simulink model "SVPWM"  (R2015a)
settings: Solver=ode4  StartTime=0.0  StopTime=40e-3  FixedStep=Ts  RelTol=1e-3
PreLoadFcn:
  | setup;
values from neighbouring files (symbols this model uses):
  Ts = 1e-8    (= 1e-08)    [setup.m]
libraries: powerlib x5, simulink x3
settings Model: CovSFcnEnable=off  Creator=mikaczma  LastModifiedBy=Michał
settings DataIOCC: SaveOutput=off  SaveTime=off
settings DebuggingCC: SolverPrmCheckMsg=warning
settings HardwareCC: ProdHWDeviceType=ASIC/FPGA->ASIC/FPGA  TargetLongLongMode=on  TargetIntDivRoundTo=Zero  TargetEndianess=LittleEndian  TargetHWDeviceType=Generic->MATLAB Host Computer  ProdEqTarget=off

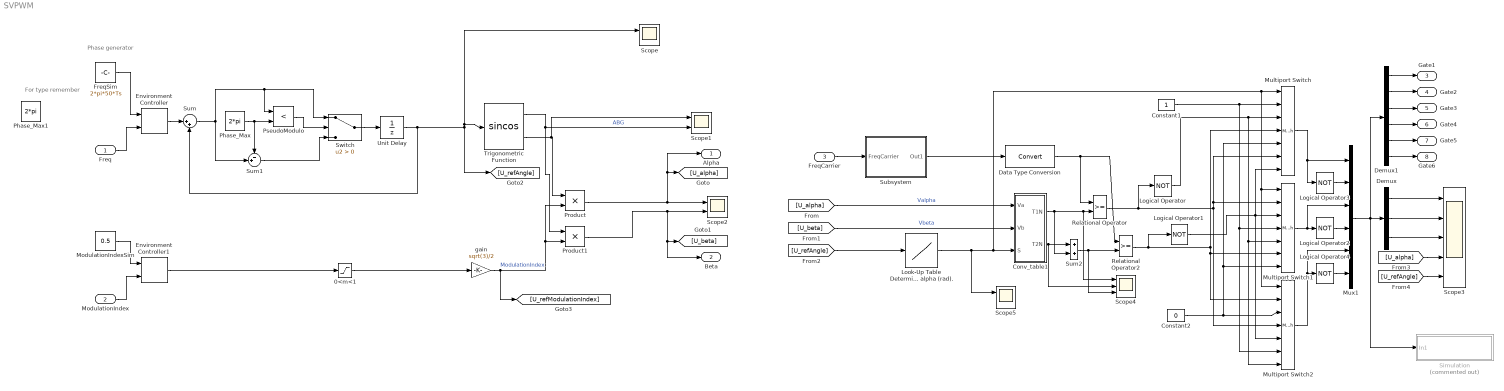
== system SVPWM ==
  note: For type remember
  note: Phase generator
  Freq : Inport
  ModulationIndex : Inport  Port=2
  FreqCarrier : Inport  Port=3
  "0<m<1 " : Saturate  UpperLimit=1  LowerLimit=0
  Constant1 : Constant  OutDataTypeStr=boolean  SampleTime=Ts
  Constant2 : Constant  Value=0  OutDataTypeStr=boolean  SampleTime=Ts
  Conv_table1 : Subsystem  VariantControl=Variant1
  Data Type Conversion : DataTypeConversion
  Demux : Demux  Outputs=[2 2 2]
  Demux1 : Demux  Outputs=6
  Environment Controller : simulink/Signal Routing/Environment Controller
  Environment Controller1 : simulink/Signal Routing/Environment Controller
  FreqSim : Constant  Value=2*pi*50*Ts  OutDataTypeStr=fixdt(1,32,24)  SampleTime=-1
  Logical Operator{,1..4} (5 alike) : Logic  Operator=NOT  OutDataTypeStr=boolean
  "Look-Up Table Determine the sector of U* based on alpha (rad). " : Lookup  InputValues=[0:pi/3:5*pi/3]  Table=[1:6]  LookUpMeth=Use Input Below  SaturateOnIntegerOverflow=on
  ModulationIndexSim : Constant  Value=0.5  OutDataTypeStr=fixdt(1,32,24)  SampleTime=-1
  Multiport Switch : MultiPortSwitch  Inputs=6  SaturateOnIntegerOverflow=on  InputSameDT=on
  Multiport Switch1 : MultiPortSwitch  Inputs=6  SaturateOnIntegerOverflow=on  InputSameDT=on
  Multiport Switch2 : MultiPortSwitch  Inputs=6  SaturateOnIntegerOverflow=on  InputSameDT=on
  Mux1 : Mux  Inputs=6
  Phase_Max : Constant  Value=2*pi  OutDataTypeStr=fixdt(1,32,24)  SampleTime=-1
  Phase_Max1 : Constant  Value=2*pi  OutDataTypeStr=fixdt(1,32,24)  SampleTime=-1
  Product : Product  OutMin=-2  OutMax=2  OutDataTypeStr=fixdt(1,64,60)
  Product1 : Product  OutMin=-2  OutMax=2  OutDataTypeStr=fixdt(1,64,60)
  PseudoModulo : RelationalOperator  Operator=<  OutDataTypeStr=boolean
  Relational Operator : RelationalOperator  OutDataTypeStr=boolean  InputSameDT=on
  Relational Operator2 : RelationalOperator  OutDataTypeStr=boolean  InputSameDT=on
  Scope{,1..2,5} (4 alike) : Scope  NumInputPorts=2
      Scope settings: YMin=0.075~-1  YMax=0.135~1
      Scope1 settings: YMin=-1~-1  YMax=1~1
      Scope2 settings: YMin=-0.45~-0.45  YMax=0.45~0.45  SaveName=ScopeData2
      Scope5 settings: YMin=0.2~-1  YMax=0.4~1  SaveName=ScopeData5
  Scope3 : Scope  NumInputPorts=5
      settings: YMin=0~0~0~-0.4~0  YMax=1~1~1~0.5~2.5  SaveName=ScopeData3
  Scope4 : Scope  NumInputPorts=3
      settings: YMin=-1~-0.5~-5  YMax=0.4~1~5  SaveName=ScopeData4
  Simulation : Subsystem  Commented=on
  Subsystem : Subsystem
  Sum : Sum  Inputs=|++  OutDataTypeStr=Inherit: Same as first input
  Sum1 : Sum  Inputs=-+|  OutMin=0  OutMax=2*pi  OutDataTypeStr=Inherit: Same as first input
  Sum2 : Sum  SaturateOnIntegerOverflow=on  InputSameDT=on  OutDataTypeStr=Inherit: Same as first input
  Switch : Switch  Criteria=u2 > Threshold
  Trigonometric Function : Trigonometry  Operator=sincos  ApproximationMethod=CORDIC  NumberOfIterations=20
  Unit Delay : UnitDelay  SampleTime=-1
  gain : Gain  Gain=sqrt(3)/2  OutDataTypeStr=fixdt(1,32,30)  SaturateOnIntegerOverflow=on  ParamDataTypeStr=Inherit: Same as input
  Alpha : Outport  OutMin=-2  OutMax=2
  Beta : Outport  Port=2  OutMin=-2  OutMax=2
  Gate1 : Outport  Port=3  OutDataTypeStr=boolean
  Gate2 : Outport  Port=4  OutDataTypeStr=boolean
  Gate3 : Outport  Port=5  OutDataTypeStr=boolean
  Gate4 : Outport  Port=6  OutDataTypeStr=boolean
  Gate5 : Outport  Port=7  OutDataTypeStr=boolean
  Gate6 : Outport  Port=8  OutDataTypeStr=boolean
  wires:
  Sum/1 -> Sum1/2, PseudoModulo/1, Switch/1
  Unit Delay/1 -> Trigonometric Function/1, Scope/1, [U_refAngle], Sum/2
  Phase_Max/1 -> PseudoModulo/2, Sum1/1
  PseudoModulo/1 -> Switch/2
  Switch/1 -> Unit Delay/1
  Sum1/1 -> Switch/3
  Environment Controller/1 -> Sum/1
  Freq/1 -> Environment Controller/2
  FreqSim/1 -> Environment Controller/1
  Trigonometric Function/2 -> Scope1/1, Product/1
  ModulationIndex/1 -> Environment Controller1/2
  ModulationIndexSim/1 -> Environment Controller1/1
  Environment Controller1/1 -> "0<m<1 "/1
  Trigonometric Function/1 -> Product1/1, Scope1/2  "ABG"
  "0<m<1 "/1 -> gain/1
  Subsystem/1(Out1) -> Data Type Conversion/1
  [U_beta] -> Conv_table1/2(Vb)  "Vbeta"
  [U_alpha] -> Conv_table1/1(Va)  "Valpha"
  Constant2/1 -> Multiport Switch1/7, Multiport Switch/5, Multiport Switch2/3
  Logical Operator1/1 -> Multiport Switch/7, Multiport Switch2/5, Multiport Switch1/3
  Logical Operator/1 -> Multiport Switch2/7, Multiport Switch1/5, Multiport Switch/3
  Relational Operator2/1 -> Multiport Switch1/6, Multiport Switch2/2, Multiport Switch/4, Logical Operator1/1
  Relational Operator/1 -> Multiport Switch/6, Multiport Switch1/2, Multiport Switch2/4, Logical Operator/1
  Constant1/1 -> Multiport Switch2/6, Multiport Switch1/4, Multiport Switch/2
  Sum2/1 -> Scope4/3, Relational Operator2/2
  Conv_table1/2(T2N) -> Scope4/2, Sum2/1
  Conv_table1/1(T1N) -> Sum2/2, Scope4/1, Relational Operator/2
  Logical Operator3/1 -> Mux1/2
  Logical Operator2/1 -> Mux1/4
  Logical Operator4/1 -> Mux1/6
  Multiport Switch/1 -> Logical Operator3/1, Mux1/1
  Multiport Switch1/1 -> Logical Operator2/1, Mux1/3
  Multiport Switch2/1 -> Mux1/5, Logical Operator4/1
  "Look-Up Table Determine the sector of U* based on alpha (rad). "/1 -> Scope5/1, Conv_table1/3(S), Multiport Switch2/1, Multiport Switch1/1, Multiport Switch/1
  Product/1 -> Alpha/1, [U_alpha], Scope2/1
  Product1/1 -> Beta/1, [U_beta], Scope2/2
  gain/1 -> [U_refModulationIndex], Product1/2, Product/2  "ModulationIndex"
  [U_refAngle] -> "Look-Up Table Determine the sector of U* based on alpha (rad). "/1
  Demux/2 -> Scope3/2
  Demux/1 -> Scope3/1
  Demux/3 -> Scope3/3
  [U_alpha] -> Scope3/4
  [U_refAngle] -> Scope3/5
  Mux1/1 -> Demux1/1, Simulation/1(In1), Demux/1
  Data Type Conversion/1 -> Relational Operator/1, Relational Operator2/1
  Demux1/1 -> Gate1/1
  Demux1/4 -> Gate4/1
  Demux1/3 -> Gate3/1
  Demux1/2 -> Gate2/1
  Demux1/5 -> Gate5/1
  Demux1/6 -> Gate6/1
  FreqCarrier/1 -> Subsystem/1(FreqCarrier)

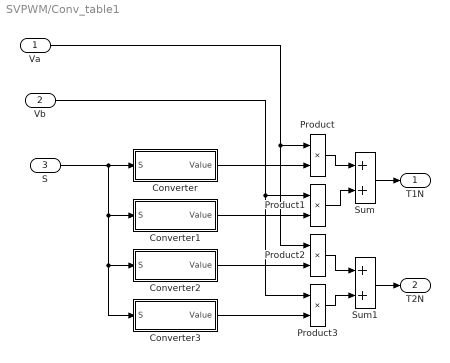
== system SVPWM/Conv_table1 ==
  Va : Inport
  Vb : Inport  Port=2
  S : Inport  Port=3
  Converter : Subsystem  VariantControl=Variant1  mask{Data=[1 1 0 -1 -1 0]}
      mask prompts: Data "Data Coefficients"
      mask Display:
      | port_label('input', 1, 'Sector')
      | port_label('output', 1, 'Value')
  Converter1 : Subsystem  VariantControl=Variant1  mask{Data=[-1/sqrt(3) 1/sqrt(3) 2/sqrt(3) 1/sqrt(3) -1/sqrt(3) -2/sqrt(3)]}
      mask prompts: Data "Data Coefficients"
      mask Display:
      | port_label('input', 1, 'Sector')
      | port_label('output', 1, 'Value')
  Converter2 : Subsystem  VariantControl=Variant1  mask{Data=[0 -1 -1 0 1 1]}
      mask prompts: Data "Data Coefficients"
      mask Display:
      | port_label('input', 1, 'Sector')
      | port_label('output', 1, 'Value')
  Converter3 : Subsystem  VariantControl=Variant1  mask{Data=[2/sqrt(3) 1/sqrt(3) -1/sqrt(3) -2/sqrt(3) -1/sqrt(3) 1/sqrt(3)]}
      mask prompts: Data "Data Coefficients"
      mask Display:
      | port_label('input', 1, 'Sector')
      | port_label('output', 1, 'Value')
  Product{,1..3} (4 alike) : Product  SaturateOnIntegerOverflow=on  InputSameDT=on  OutDataTypeStr=Inherit: Same as first input
  Sum : Sum  SaturateOnIntegerOverflow=on  InputSameDT=on  OutDataTypeStr=Inherit: Same as first input
  Sum1 : Sum  SaturateOnIntegerOverflow=on  InputSameDT=on  OutDataTypeStr=Inherit: Same as first input
  T1N : Outport
  T2N : Outport  Port=2
  wires:
  Va/1 -> Product/1, Product2/1
  Converter/1(Value) -> Product/2
  Vb/1 -> Product1/1, Product3/1
  Converter1/1(Value) -> Product1/2
  Converter2/1(Value) -> Product2/2
  Converter3/1(Value) -> Product3/2
  Product/1 -> Sum/1
  Product1/1 -> Sum/2
  Product2/1 -> Sum1/1
  Product3/1 -> Sum1/2
  Sum/1 -> T1N/1
  Sum1/1 -> T2N/1
  S/1 -> Converter3/1(S), Converter2/1(S), Converter1/1(S), Converter/1(S)

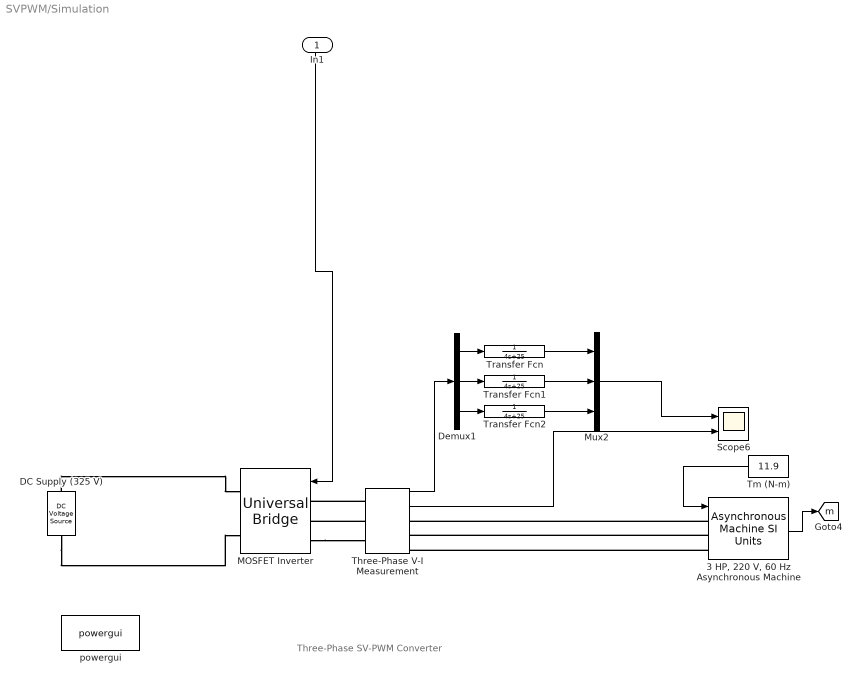
== system SVPWM/Simulation ==
  note: Three-Phase SV-PWM Converter
  In1 : Inport
  "3 HP, 220 V, 60 Hz Asynchronous Machine" : powerlib/Machines/Asynchronous Machine SI Units  RotorType=Squirrel-cage  PresetModel=No  MechanicalLoad=Torque Tm  ShowDetailedParameters=on  ReferenceFrame=Stationary  Units=SI  MeasurementBus=off  NominalParameters=[ 3*746, 220, 60 ]  Stator="[ 0.435  2*2.0e-3 ]"  Rotor="[ 0.816  2.0e-3 ]"  Cage1=[ 0.022 0.226/377]  Cage2=[ 0.022 0.226/377]  Lm=69.31e-3  Mechanical="[ 0.089  0  2 ]"  PolePairs=2  InitialConditions=[0.044533 0 11.138 11.138 11.138 -39.6 -159.6 80.4]  SimulateSaturation=off  Saturation=[0 0;0 0]  LoadFlowParameters=2000  TsPowergui=0  TsBlock=-1  IterativeModel=Trapezoidal non iterative  Pmec=0
  DC Supply (325 V) : powerlib/Electrical Sources/DC Voltage Source  Amplitude=325  Measurements=None
  Demux1 : Demux  Outputs=3
  MOSFET Inverter : powerlib/Power Electronics/Universal Bridge  Arms=3  SnubberResistance=1e5  SnubberCapacitance=inf  Device=MOSFET / Diodes  Ron=0.2e-3  Lon=0  ForwardVoltages="[  0  0  ]"  ForwardVoltage=0  GTOparameters=[ 10e-6 , 20e-6 ]  IGBTparameters=[ 1e-6 , 2e-6 ]  Measurements=None  Measurements_2=None  converterType=Rectifier
  Mux2 : Mux  Inputs=3
  Scope6 : Scope  NumInputPorts=2
      settings: YMin=-0.2~-60  YMax=0.3~90  SaveName=ScopeData6
  Three-Phase V-I Measurement : powerlib/Measurements/Three-Phase V-I Measurement  VoltageMeasurement=phase-to-phase  SetLabelV=off  LabelV=Vabc  Vpu=off  VpuLL=off  CurrentMeasurement=yes  SetLabelI=off  LabelI=Iabc  Ipu=off  Pbase=100e6  Vbase=500e3  OutputType=Complex  PhasorSimulation=off  PSBequivalent=0
  Tm (N-m) : Constant  Value=11.9
  Transfer Fcn : TransferFcn  Denominator=[4 25]
  Transfer Fcn1 : TransferFcn  Denominator=[4 25]
  Transfer Fcn2 : TransferFcn  Denominator=[4 25]
  powergui : powerlib/powergui  Priority=2  SimulationMode=Discrete  SolverType=Tustin/Backward Euler (TBE)  SampleTime=Ts  frequency=60  SPID=off  DisableSnubberDevices=off  DisableRonSwitches=off  DisableVfSwitches=off  SwTol=0  DisplayEquations=off  Interpol=off  methode=off  Ts=0  FunctionMessages=off  echomessages=off  HookPort=off  EnableUseOfTLC=off  x0status=blocks  frequencyindice=60  Pbase=100e6  ErrMax=1e-4  Iterations=50  UnitsV=kV  UnitsW=MW  buscounter=0  RestoreLinks=warning  ResistiveCurrentMeasurement=off  Frange=[0:2:500]  Ylog=off  Xlog=on  ShowGrid=off  save=off  variable=ZData  structure=VI_Stator  ZoomFFT=on  StartTime=0.05  cycles=2  DisplayStyle=1  fundamental=60  FreqAxis=off  MaxFrequency=5000  frequencyindicesteady=1  RmsSteady=1  display=off
  tag scope: m=global
  wires:
  "3 HP, 220 V, 60 Hz Asynchronous Machine"/1 -> [m]
  Tm (N-m)/1 -> "3 HP, 220 V, 60 Hz Asynchronous Machine"/1
  Transfer Fcn/1 -> Mux2/1
  Transfer Fcn1/1 -> Mux2/2
  Three-Phase V-I Measurement/1 -> Demux1/1
  In1/1 -> MOSFET Inverter/1
  Transfer Fcn2/1 -> Mux2/3
  Mux2/1 -> Scope6/1
  Three-Phase V-I Measurement/2 -> Scope6/2
  Demux1/2 -> Transfer Fcn1/1
  Demux1/3 -> Transfer Fcn2/1
  Demux1/1 -> Transfer Fcn/1
  connections:
  DC Supply (325 V)/LConn1 -- MOSFET Inverter/RConn2
  DC Supply (325 V)/RConn1 -- MOSFET Inverter/RConn1
  Three-Phase V-I Measurement/LConn1 -- MOSFET Inverter/LConn1
  Three-Phase V-I Measurement/LConn2 -- MOSFET Inverter/LConn2
  "3 HP, 220 V, 60 Hz Asynchronous Machine"/LConn2 -- Three-Phase V-I Measurement/RConn2
  MOSFET Inverter/LConn3 -- Three-Phase V-I Measurement/LConn3
  "3 HP, 220 V, 60 Hz Asynchronous Machine"/LConn1 -- Three-Phase V-I Measurement/RConn1
  "3 HP, 220 V, 60 Hz Asynchronous Machine"/LConn3 -- Three-Phase V-I Measurement/RConn3

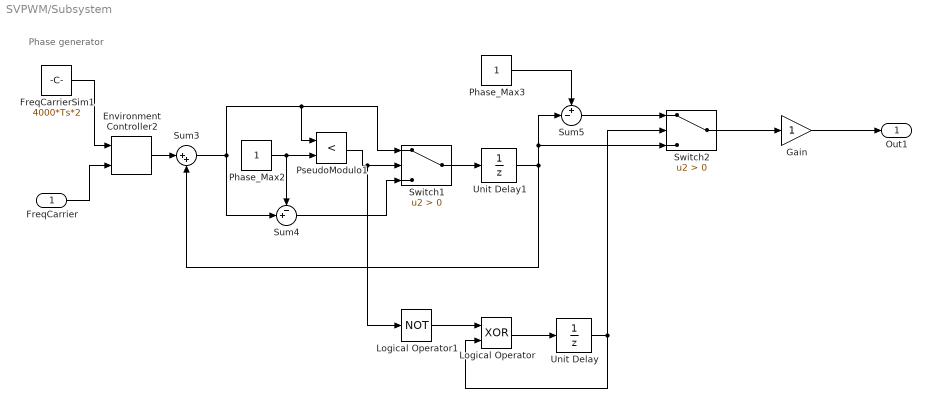
== system SVPWM/Subsystem ==
  note: Phase generator
  FreqCarrier : Inport
  Environment Controller2 : simulink/Signal Routing/Environment Controller
  FreqCarrierSim1 : Constant  Value=4000*Ts*2  OutDataTypeStr=fixdt(1,32,24)  SampleTime=-1
  Gain : Gain  OutDataTypeStr=fixdt(1,64,60)
  Logical Operator : Logic  Operator=XOR  AllPortsSameDT=off  OutDataTypeStr=boolean
  Logical Operator1 : Logic  Operator=NOT  AllPortsSameDT=off  OutDataTypeStr=boolean
  Phase_Max2 : Constant  OutDataTypeStr=fixdt(1,32,24)  SampleTime=-1
  Phase_Max3 : Constant  OutDataTypeStr=fixdt(1,32,24)  SampleTime=-1
  PseudoModulo1 : RelationalOperator  Operator=<  OutDataTypeStr=boolean
  Sum3 : Sum  Inputs=|++  OutDataTypeStr=Inherit: Same as first input
  Sum4 : Sum  Inputs=-+|  OutMin=0  OutMax=2*pi  OutDataTypeStr=Inherit: Same as first input
  Sum5 : Sum  Inputs=+-|  OutMin=0  OutMax=2*pi  OutDataTypeStr=Inherit: Same as first input
  Switch1 : Switch  Criteria=u2 > Threshold
  Switch2 : Switch  Criteria=u2 > Threshold
  Unit Delay : UnitDelay  SampleTime=-1
  Unit Delay1 : UnitDelay  SampleTime=-1
  Out1 : Outport
  wires:
  Unit Delay/1 -> Logical Operator/2, Switch2/2
  Logical Operator/1 -> Unit Delay/1
  Switch2/1 -> Gain/1
  Logical Operator1/1 -> Logical Operator/1
  FreqCarrierSim1/1 -> Environment Controller2/1
  Unit Delay1/1 -> Sum5/2, Switch2/3, Sum3/2
  Sum3/1 -> Sum4/2, PseudoModulo1/1, Switch1/1
  PseudoModulo1/1 -> Logical Operator1/1, Switch1/2
  FreqCarrier/1 -> Environment Controller2/2
  Switch1/1 -> Unit Delay1/1
  Sum4/1 -> Switch1/3
  Environment Controller2/1 -> Sum3/1
  Phase_Max2/1 -> PseudoModulo1/2, Sum4/1
  Phase_Max3/1 -> Sum5/1
  Sum5/1 -> Switch2/1
  Gain/1 -> Out1/1

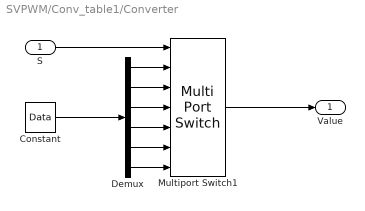
== system SVPWM/Conv_table1/Converter ==
  S : Inport
  Constant : Constant  Value=Data  OutDataTypeStr=fixdt(1,64,60)
  Demux : Demux  Outputs=6
  Multiport Switch1 : MultiPortSwitch  Inputs=6  SaturateOnIntegerOverflow=on  InputSameDT=on
  Value : Outport
  wires:
  S/1 -> Multiport Switch1/1
  Demux/1 -> Multiport Switch1/2
  Demux/2 -> Multiport Switch1/3
  Demux/3 -> Multiport Switch1/4
  Demux/4 -> Multiport Switch1/5
  Demux/5 -> Multiport Switch1/6
  Demux/6 -> Multiport Switch1/7
  Constant/1 -> Demux/1
  Multiport Switch1/1 -> Value/1

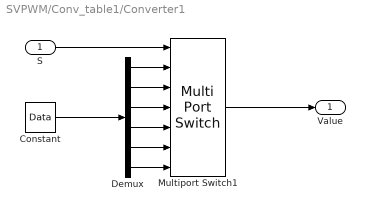
== system SVPWM/Conv_table1/Converter1 ==
  S : Inport
  Constant : Constant  Value=Data  OutDataTypeStr=fixdt(1,64,60)
  Demux : Demux  Outputs=6
  Multiport Switch1 : MultiPortSwitch  Inputs=6  SaturateOnIntegerOverflow=on  InputSameDT=on
  Value : Outport
  wires:
  Multiport Switch1/1 -> Value/1
  Constant/1 -> Demux/1
  Demux/6 -> Multiport Switch1/7
  Demux/5 -> Multiport Switch1/6
  Demux/4 -> Multiport Switch1/5
  Demux/3 -> Multiport Switch1/4
  Demux/2 -> Multiport Switch1/3
  Demux/1 -> Multiport Switch1/2
  S/1 -> Multiport Switch1/1

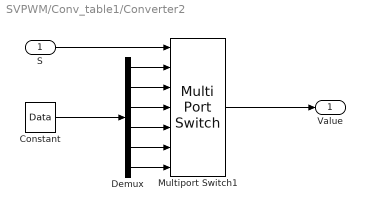
== system SVPWM/Conv_table1/Converter2 ==
  S : Inport
  Constant : Constant  Value=Data  OutDataTypeStr=fixdt(1,64,60)
  Demux : Demux  Outputs=6
  Multiport Switch1 : MultiPortSwitch  Inputs=6  SaturateOnIntegerOverflow=on  InputSameDT=on
  Value : Outport
  wires:
  S/1 -> Multiport Switch1/1
  Demux/1 -> Multiport Switch1/2
  Demux/2 -> Multiport Switch1/3
  Demux/3 -> Multiport Switch1/4
  Demux/4 -> Multiport Switch1/5
  Demux/5 -> Multiport Switch1/6
  Demux/6 -> Multiport Switch1/7
  Constant/1 -> Demux/1
  Multiport Switch1/1 -> Value/1

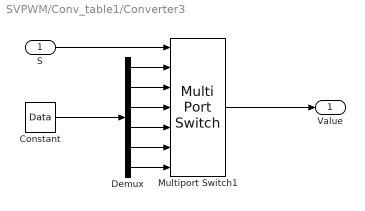
== system SVPWM/Conv_table1/Converter3 ==
  S : Inport
  Constant : Constant  Value=Data  OutDataTypeStr=fixdt(1,64,60)
  Demux : Demux  Outputs=6
  Multiport Switch1 : MultiPortSwitch  Inputs=6  SaturateOnIntegerOverflow=on  InputSameDT=on
  Value : Outport
  wires:
  Multiport Switch1/1 -> Value/1
  Constant/1 -> Demux/1
  Demux/6 -> Multiport Switch1/7
  Demux/5 -> Multiport Switch1/6
  Demux/4 -> Multiport Switch1/5
  Demux/3 -> Multiport Switch1/4
  Demux/2 -> Multiport Switch1/3
  Demux/1 -> Multiport Switch1/2
  S/1 -> Multiport Switch1/1
